simulink model "extinterrupt"  (R2022b)
settings: Solver=FixedStepDiscrete  StartTime=0.0  StopTime=inf  FixedStep=0.001  RelTol=1e-3
libraries: teensy_lib x2
settings Model: Creator=LabUser  LastModifiedBy=LabUser
settings OptimizationCC: EnhancedBackFolding=on  PassReuseOutputArgsAs=Individual arguments  ZeroExternalMemoryAtStartup=off  ZeroInternalMemoryAtStartup=off  OptimizeBlockOrder=speed  DifferentSizesBufferReuse=on  OptimizationCustomize=off  EfficientTunableParamExpr=on
settings DebuggingCC: ParameterTunabilityLossMsg=error
settings HardwareCC: ProdBitPerPointer=32  ProdBitPerSizeT=32  ProdBitPerPtrDiffT=32  ProdLargestAtomicInteger=Long  ProdLargestAtomicFloat=Double  ProdWordSize=32  ProdHWDeviceType=ARM Compatible->ARM Cortex-M
settings SFSimCC: MATLABDynamicMemAlloc=off
settings RTWCC: Description=Teensy ERT Target  SystemTargetFile=teensy_ert.tlc  TemplateMakefile=teensy_ert.tmf  TargetLang=C++
settings CodeAppCC: ForceParamTrailComments=on  IgnoreCustomStorageClasses=off  OperatorAnnotations=on  SimulinkDataObjDesc=on  SFDataObjDesc=on  InsertBlockDesc=on
settings STFCustomTargetCC: TargetLibSuffix=.a  TargetLangStandard=C++11 (ISO)  MultiwordLength=256  GenerateSampleERTMain=on  CombineOutputUpdateFcns=on  ERTCustomFileBanners=on  SupportContinuousTime=off  SupportNonInlinedSFcns=off  RemoveResetFunc=on  MATLABClassNameForMDSCustomization=Simulink.SoftwareTarget.ERTCustomization  CPPClassGenCompliant=on  SystemTargetFile=teensy_ert.tlc
settings ERTTargetCC: TargetLangStandard=C++11 (ISO)  GenerateSampleERTMain=on  ParMdlRefBuildCompliant=off  CompOptLevelCompliant=off  ConcurrentExecutionCompliant=off  ModelStepFunctionPrototypeControlCompliant=off  UseToolchainInfoCompliant=off  ExtModeTransport=1  ExtModeMexFile=ext_serial_win32_comm  ExtModeMexArgs=0 7 4000000  ERTCustomFileTemplate=teensy_ert_file_process.tlc

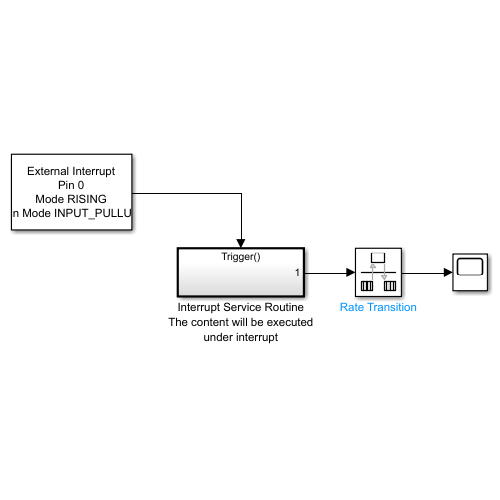
[thumbnail: Simulink's stored preview of the top-level diagram]
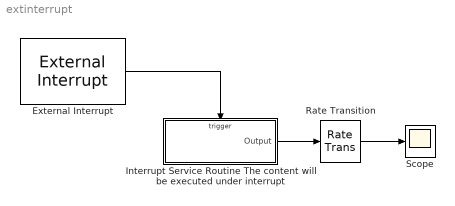
== system extinterrupt ==
  External Interrupt : teensy_lib/External Interrupt  Mode=RISING  Prio=20  Pinmode=INPUT_PULLUP  Pin=0  Simulation=off  Timer=off
      settings: LibrarySourceBlock=arduino_lib/External Interrupt
  Interrupt Service Routine The content will be executed under interrupt : Subsystem  TreatAsAtomicUnit=on
  Rate Transition : RateTransition  Deterministic=off
  Scope : Scope
  wires:
  External Interrupt/1 -> Interrupt Service Routine The content will be executed under interrupt/Trigger
  Interrupt Service Routine The content will be executed under interrupt/1(Output) -> Rate Transition/1
  Rate Transition/1 -> Scope/1

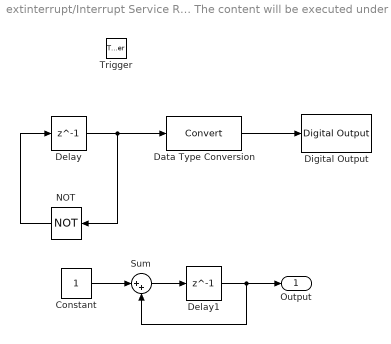
== system extinterrupt/Interrupt Service Routine The content will be executed under interrupt ==
  Trigger : TriggerPort  TriggerType=function-call  VariantControl=(inherit)
  Constant : Constant  OutDataTypeStr=int32  SampleTime=-1
  Data Type Conversion : DataTypeConversion  SaturateOnIntegerOverflow=off  RndMeth=Floor
  Delay : Delay  DelayLength=1  InitialCondition=0
  Delay1 : Delay  DelayLength=1  InitialCondition=0
  Digital Output : teensy_lib/Digital Output  SParameter1=13  SampleTime=-1
  NOT : Logic  Operator=NOT  IconShape=distinctive  AllPortsSameDT=off  OutDataTypeStr=boolean
  Sum : Sum  Inputs=|++
  Output : Outport
  wires:
  Delay/1 -> NOT/1, Data Type Conversion/1
  Delay1/1 -> Sum/2, Output/1
  NOT/1 -> Delay/1
  Data Type Conversion/1 -> Digital Output/1
  Sum/1 -> Delay1/1
  Constant/1 -> Sum/1
